simulink model "helikopter_maketa"  (Simulink 7.7)
settings: Solver=ode45  StartTime=0.0  StopTime=5  RelTol=1e-3
values from neighbouring files (symbols this model uses):
  bh = 0.05    [helikopter_maketa_paraametri.m]    (also in helikopter_maketa_parametri.m)
  bv = 0.05    [helikopter_maketa_paraametri.m]    (also in helikopter_maketa_parametri.m)
  dz1_z = 0.07    [helikopter_maketa_paraametri.m]    (also in helikopter_maketa_parametri.m)
  dz2_z = 0.08    [helikopter_maketa_paraametri.m]    (also in helikopter_maketa_parametri.m)
  g = 9.81    [helikopter_maketa_paraametri.m]    (also in helikopter_maketa_parametri.m)
  I = m1*l1^2 + m2*l2^2 + m3*l3^2    (= 0.0128174)    [helikopter_maketa_paraametri.m]    (also in helikopter_maketa_parametri.m)
  K1_u = 0.14/l1    (= 0.474576271186)    [helikopter_maketa_paraametri.m]    (also in helikopter_maketa_parametri.m)
  K1_z = 0.014*l1/l2    (= 0.01475)    [helikopter_maketa_paraametri.m]    (also in helikopter_maketa_parametri.m)
  K2_z = 0.05    [helikopter_maketa_paraametri.m]    (also in helikopter_maketa_parametri.m)
  l1 = 0.295    [helikopter_maketa_paraametri.m]    (also in helikopter_maketa_parametri.m)
  l2 = 0.280    (= 0.28)    [helikopter_maketa_paraametri.m]    (also in helikopter_maketa_parametri.m)
  l3 = 0.120    (= 0.12)    [helikopter_maketa_paraametri.m]    (also in helikopter_maketa_parametri.m)
  m1 = 0.120    (= 0.12)    [helikopter_maketa_paraametri.m]    (also in helikopter_maketa_parametri.m)
  m2 = 0.020    (= 0.02)    [helikopter_maketa_paraametri.m]    (also in helikopter_maketa_parametri.m)
  m3 = 0.056    [helikopter_maketa_paraametri.m]    (also in helikopter_maketa_parametri.m)
  theta0 = -5*pi/180    (= -0.0872664625997)    [helikopter_maketa_paraametri.m]    (also in helikopter_maketa_parametri.m = -0.872664625997)
  theta_max = 50*pi/180    (= 0.872664625997)    [helikopter_maketa_paraametri.m]    (also in helikopter_maketa_parametri.m)
  theta_min = -50*pi/180    (= -0.872664625997)    [helikopter_maketa_paraametri.m]    (also in helikopter_maketa_parametri.m)
  u1_max = 12    [helikopter_maketa_paraametri.m]    (also in helikopter_maketa_parametri.m)
  u1_min = 0    [helikopter_maketa_paraametri.m]    (also in helikopter_maketa_parametri.m)
  u2_max = 5    [helikopter_maketa_paraametri.m]    (also in helikopter_maketa_parametri.m)
  u2_min = -5    [helikopter_maketa_paraametri.m]    (also in helikopter_maketa_parametri.m)
settings Model: Creator=damjan  LastModifiedBy=Damjan
settings DebuggingCC: SolverPrmCheckMsg=none  FcnCallInpInsideContextMsg=Enable All
settings GRTTargetCC: CombineOutputUpdateFcns=on

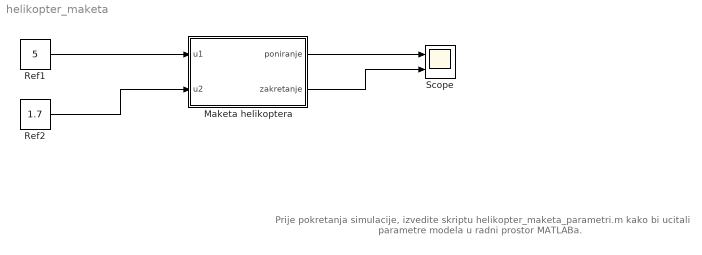
== system helikopter_maketa ==
  note: Prije pokretanja simulacije, izvedite skriptu
      | helikopter_maketa_parametri.m kako bi
      | ucitali parametre modela u radni prostor
      | MATLABa.
  Maketa helikoptera : Subsystem
  Ref1 : Constant  Value=5
  Ref2 : Constant  Value=1.7
  Scope : Scope  NumInputPorts=2
      settings: YMin=-0.872665~-5  YMax=-0.872665~5
  wires:
  Maketa helikoptera/1(poniranje) -> Scope/1
  Maketa helikoptera/2(zakretanje) -> Scope/2
  Ref1/1 -> Maketa helikoptera/1(u1)
  Ref2/1 -> Maketa helikoptera/2(u2)

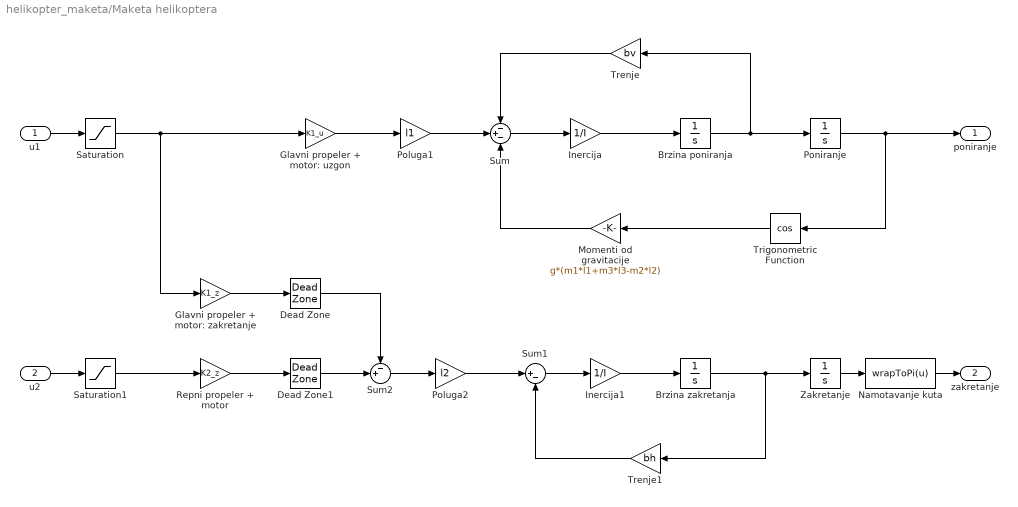
== system helikopter_maketa/Maketa helikoptera ==
  u1 : Inport
  u2 : Inport  Port=2
  Brzina poniranja : Integrator
  Brzina zakretanja : Integrator
  Dead Zone : DeadZone  LowerValue=-dz1_z  UpperValue=dz1_z  SaturateOnIntegerOverflow=on
  Dead Zone1 : DeadZone  LowerValue=-dz2_z  UpperValue=dz2_z  SaturateOnIntegerOverflow=on
  Glavni propeler + motor: uzgon : Gain  Gain=K1_u
  Glavni propeler + motor: zakretanje : Gain  Gain=K1_z
  Inercija : Gain  Gain=1/I
  Inercija1 : Gain  Gain=1/I
  Momenti od gravitacije : Gain  Gain=g*(m1*l1+m3*l3-m2*l2)
  Namotavanje kuta : MATLABFcn  MATLABFcn=wrapToPi(u)
  Poluga1 : Gain  Gain=l1
  Poluga2 : Gain  Gain=l2
  Poniranje : Integrator  InitialCondition=theta0  LimitOutput=on  UpperSaturationLimit=theta_max  LowerSaturationLimit=theta_min  ContinuousStateAttributes='theta'
  Repni propeler + motor : Gain  Gain=K2_z
  Saturation : Saturate  UpperLimit=u1_max  LowerLimit=u1_min
  Saturation1 : Saturate  UpperLimit=u2_max  LowerLimit=u2_min
  Sum : Sum  Inputs=-+-
  Sum1 : Sum  Inputs=|+-
  Sum2 : Sum  Inputs=-+|
  Trenje : Gain  Gain=bv
  Trenje1 : Gain  Gain=bh
  Trigonometric Function : Trigonometry  Operator=cos
  Zakretanje : Integrator  ContinuousStateAttributes='phi'
  poniranje : Outport
  zakretanje : Outport  Port=2
  wires:
  Inercija/1 -> Brzina poniranja/1
  Brzina poniranja/1 -> Poniranje/1, Trenje/1
  Trenje/1 -> Sum/1
  Sum/1 -> Inercija/1
  Poluga1/1 -> Sum/2
  Poniranje/1 -> Trigonometric Function/1, poniranje/1
  Trigonometric Function/1 -> Momenti od gravitacije/1
  Momenti od gravitacije/1 -> Sum/3
  Glavni propeler + motor: uzgon/1 -> Poluga1/1
  Glavni propeler + motor: zakretanje/1 -> Dead Zone/1
  Sum1/1 -> Inercija1/1
  Inercija1/1 -> Brzina zakretanja/1
  Brzina zakretanja/1 -> Zakretanje/1, Trenje1/1
  Zakretanje/1 -> Namotavanje kuta/1
  Trenje1/1 -> Sum1/2
  Repni propeler + motor/1 -> Dead Zone1/1
  Dead Zone1/1 -> Sum2/2
  Dead Zone/1 -> Sum2/1
  Sum2/1 -> Poluga2/1
  Poluga2/1 -> Sum1/1
  u2/1 -> Saturation1/1
  u1/1 -> Saturation/1
  Saturation/1 -> Glavni propeler + motor: uzgon/1, Glavni propeler + motor: zakretanje/1
  Saturation1/1 -> Repni propeler + motor/1
  Namotavanje kuta/1 -> zakretanje/1
